simulink model "seti_ct_xaui"  (Simulink 6.2)
settings: Solver=ode45  StartTime=0.0  StopTime=10  RelTol=1e-3
undefined symbols (not defined in the file): bigColBits, bigRowBits, smallColBits, smallRowBits
libraries: xbsIndex_r3 x520, xps_library x31, casper_library x10, fft_library x1
(part 2 of 4)

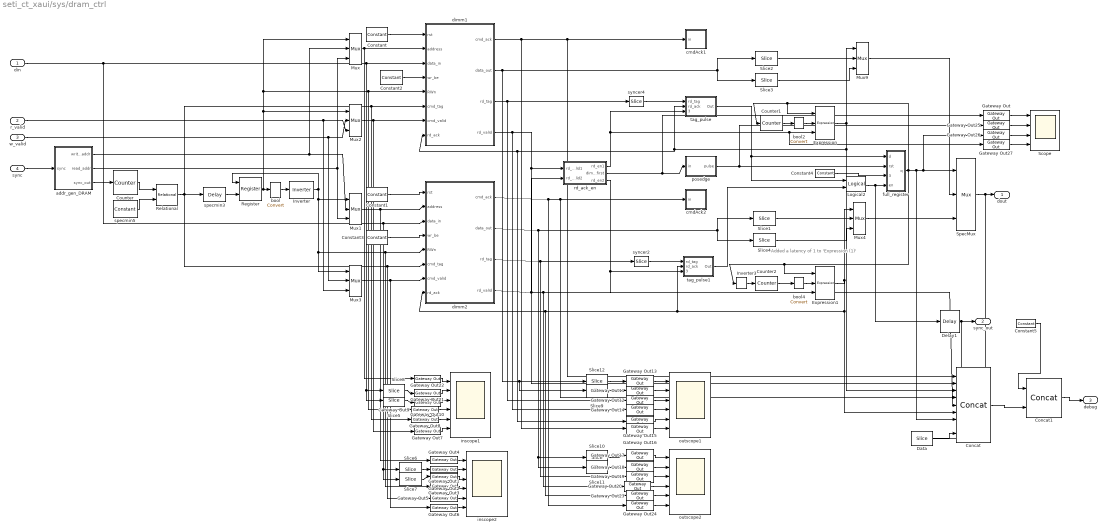
== system seti_ct_xaui/sys/dram_ctrl ==
  note: Added a latency
      | of 1 to 'Expression (1)'
  din : Inport  Port=1  LatchInput=off
  r_valid : Inport  Port=2  LatchInput=off
  w_valid : Inport  Port=3  LatchInput=off
  sync : Inport  Port=4  LatchInput=off
  Concat : xbsIndex_r3/Concat  num_inputs=9  explicit_period=off  period=1  dbl_ovrd=off
  Concat1 : xbsIndex_r3/Concat  num_inputs=2  explicit_period=off  period=1  dbl_ovrd=off
  Constant : xbsIndex_r3/Constant  const=0  equ=P=C  arith_type=Boolean  n_bits=1  bin_pt=0  opselect=C  inp2=PCIN>>17  opr=+  inp1=P  carry=CIN  iostate=0  explicit_period=on  period=1  dbl_ovrd=off
  Constant1 : xbsIndex_r3/Constant  const=0  equ=P=C  arith_type=Boolean  n_bits=1  bin_pt=0  opselect=C  inp2=PCIN>>17  opr=+  inp1=P  carry=CIN  iostate=0  explicit_period=on  period=1  dbl_ovrd=off
  Constant2 : xbsIndex_r3/Constant  const=2^18-1  equ=P=C  arith_type=Unsigned  n_bits=18  bin_pt=0  opselect=C  inp2=PCIN>>17  opr=+  inp1=P  carry=CIN  iostate=0  explicit_period=on  period=1  dbl_ovrd=off
  Constant3 : xbsIndex_r3/Constant  const=2^18-1  equ=P=C  arith_type=Unsigned  n_bits=18  bin_pt=0  opselect=C  inp2=PCIN>>17  opr=+  inp1=P  carry=CIN  iostate=0  explicit_period=on  period=1  dbl_ovrd=off
  Constant4 : xbsIndex_r3/Constant  const=0  equ=P=C  arith_type=Boolean  n_bits=1  bin_pt=0  opselect=C  inp2=PCIN>>17  opr=+  inp1=P  carry=CIN  iostate=0  explicit_period=off  period=1  dbl_ovrd=off
  Constant5 : xbsIndex_r3/Constant  const=0  equ=P=C  arith_type=Unsigned  n_bits=8  bin_pt=0  opselect=C  inp2=PCIN>>17  opr=+  inp1=P  carry=CIN  iostate=0  explicit_period=off  period=1  dbl_ovrd=off
  Counter : xbsIndex_r3/Counter  cnt_type=Free Running  n_bits=spec_len + num_spec  bin_pt=0  arith_type=Unsigned  start_count=0  cnt_to=Inf  cnt_by_val=1  operation=Up  explicit_period=off  period=1  load_pin=off  rst=on  en=off  dbl_ovrd=off  show_param=off  use_rpm=on  gen_core=off
      settings: xl_area=[0, 0, 0, 0, 0, 0, 0]
  Counter1 : xbsIndex_r3/Counter  cnt_type=Free Running  n_bits=1  bin_pt=0  arith_type=Unsigned  start_count=0  cnt_to=Inf  cnt_by_val=1  operation=Up  explicit_period=off  period=1  load_pin=off  rst=on  en=off  dbl_ovrd=off  show_param=off  use_rpm=on  gen_core=off
      settings: xl_area=[0, 0, 0, 0, 0, 0, 0]
  Counter2 : xbsIndex_r3/Counter  cnt_type=Free Running  n_bits=1  bin_pt=0  arith_type=Unsigned  start_count=0  cnt_to=Inf  cnt_by_val=1  operation=Up  explicit_period=off  period=1  load_pin=off  rst=on  en=off  dbl_ovrd=off  show_param=off  use_rpm=on  gen_core=off
      settings: xl_area=[0, 0, 0, 0, 0, 0, 0]
  Data : xbsIndex_r3/Slice  mode=Lower Bit Location + Width  nbits=16  bit1=0  base1=MSB of Input  bit0=0  base0=LSB of Input  boolean_output=off  explicit_period=off  period=1  dbl_ovrd=off
  Delay1 : xbsIndex_r3/Delay  latency=1  reg_retiming=off  explicit_period=off  period=1  en=off  accept_only_valid=off  init_zero=on  dbl_ovrd=off  show_param=off
      settings: xl_area=[0, 0, 0, 0, 0, 0, 0]
  Expression : xbsIndex_r3/Expression  expression=~a & b & c  precision=Full  arith_type=Unsigned  n_bits=8  bin_pt=2  align_bp=on  latency=1  explicit_period=off  period=1  en=off  dbl_ovrd=off  show_param=off
      settings: xl_area=[0, 0, 0, 0, 0, 0, 0]
  Expression1 : xbsIndex_r3/Expression  expression=a & b & c  precision=Full  arith_type=Unsigned  n_bits=8  bin_pt=2  align_bp=on  latency=1  explicit_period=off  period=1  en=off  dbl_ovrd=off  show_param=off
      settings: xl_area=[0, 0, 0, 0, 0, 0, 0]
  Gateway Out{,25..27} (4 alike) : xbsIndex_r3/Gateway Out  output_type=Double  nbits=8  bin_pt=6  arith_type=Boolean  quantization=Truncate  overflow=Wrap  hdl_port=on  timing_constraint=None  locs_specified=off  LOCs={}  needs_fixed_name=off  show_param=off
      settings: xl_area=[0, 0, 0, 0, 0, 0, 0]
  Gateway Out{1..24} (24 alike) : xbsIndex_r3/Gateway Out  output_type=Double  nbits=8  bin_pt=6  arith_type=Boolean  quantization=Truncate  overflow=Wrap  hdl_port=off  timing_constraint=None  locs_specified=off  LOCs={}  needs_fixed_name=off  show_param=off
      settings: xl_area=[0, 0, 0, 0, 0, 0, 0]
  Inverter : xbsIndex_r3/Inverter  latency=0  explicit_period=off  period=1  en=off  dbl_ovrd=off  show_param=off
      settings: xl_area=[0, 0, 0, 0, 0, 0, 0]
  Inverter3 : xbsIndex_r3/Inverter  latency=0  explicit_period=off  period=1  en=off  dbl_ovrd=off  show_param=off
      settings: xl_area=[0, 0, 0, 0, 0, 0, 0]
  Logical2 : xbsIndex_r3/Logical  logical_function=OR  inputs=2  precision=Full  arith_type=Unsigned  n_bits=8  bin_pt=2  align_bp=on  latency=0  explicit_period=off  period=1  en=off  dbl_ovrd=off  show_param=off
      settings: xl_area=[0, 0, 0, 0, 0, 0, 0]
  Mux{,1..4,9} (6 alike) : xbsIndex_r3/Mux  inputs=2  precision=Full  arith_type="Signed  (2's comp)"  n_bits=8  bin_pt=2  quantization=Truncate  overflow=Wrap  latency=0  explicit_period=off  period=1  en=off  dbl_ovrd=off  show_param=off  mux_type=off  use_rpm=off  gen_core=off
      settings: xl_area=[0, 0, 0, 0, 0, 0, 0]
  Register : xbsIndex_r3/Register  init=0  reg_only_valid=off  explicit_period=off  period=1  rst=off  en=on  out_en=off  dbl_ovrd=off  show_param=off
      settings: xl_area=[0, 0, 0, 0, 0, 0, 0]
  Relational : xbsIndex_r3/Relational  mode=a=b  latency=1  explicit_period=off  period=1  en=off  dbl_ovrd=off  show_param=off
      settings: xl_area=[0, 0, 0, 0, 0, 0, 0]
  Scope : Scope  NumInputPorts=4
      settings: YMin=-5~-5~-5~-5  YMax=5~5~5~5  SaveName=ScopeData11
  Slice{1..2,5,7,9,11} (6 alike) : xbsIndex_r3/Slice  mode=Lower Bit Location + Width  nbits=72  bit1=0  base1=MSB of Input  bit0=0  base0=LSB of Input  boolean_output=off  explicit_period=off  period=1  dbl_ovrd=off
  Slice{3..4,6,8,10,12} (6 alike) : xbsIndex_r3/Slice  mode=Upper Bit Location + Width  nbits=72  bit1=0  base1=MSB of Input  bit0=0  base0=LSB of Input  boolean_output=off  explicit_period=off  period=1  dbl_ovrd=off
  SpecMux : xbsIndex_r3/Mux  inputs=2  precision=Full  arith_type="Signed  (2's comp)"  n_bits=8  bin_pt=2  quantization=Truncate  overflow=Wrap  latency=1  explicit_period=off  period=1  en=off  dbl_ovrd=off  show_param=off  mux_type=off  use_rpm=off  gen_core=off
      settings: xl_area=[0, 0, 0, 0, 0, 0, 0]
  addr_gen_DRAM : Subsystem  mask{numSpecs=2^num_spec, length=2^spec_len}
      mask prompts: numSpecs "Number of Spectrums?"; length "Length of Spectrum?"
      mask init:
      | address_gen_dram_mask;
  bool : xbsIndex_r3/Convert  arith_type=Boolean  n_bits=8  bin_pt=6  quantization=Truncate  overflow=Wrap  latency=0  explicit_period=on  period=1  dbl_ovrd=off  show_param=off  inserted_by_tool=off  pipeline=off
      settings: xl_area=[0, 0, 0, 0, 0, 0, 0]
  bool2 : xbsIndex_r3/Convert  arith_type=Boolean  n_bits=8  bin_pt=6  quantization=Truncate  overflow=Wrap  latency=0  explicit_period=on  period=1  dbl_ovrd=off  show_param=off  inserted_by_tool=off  pipeline=off
      settings: xl_area=[0, 0, 0, 0, 0, 0, 0]
  bool4 : xbsIndex_r3/Convert  arith_type=Boolean  n_bits=8  bin_pt=6  quantization=Truncate  overflow=Wrap  latency=0  explicit_period=on  period=1  dbl_ovrd=off  show_param=off  inserted_by_tool=off  pipeline=off
      settings: xl_area=[0, 0, 0, 0, 0, 0, 0]
  cmdAck1 : Subsystem
  cmdAck2 : Subsystem
  dimm1 : Subsystem  Tag=xps:dram  AncestorBlock=xps_library/dram  mask(dram){dimm=1, arith_type=Unsigned, bin_pt=0, ip_clock=200, sample_period=1, use_sim=on, bank_mgt=off, wide_data=off, half_burst=off}
      mask prompts: arith_type "Data Type"; bin_pt "Data binary point"; ip_clock "Datapath clock rate (MHz)"; sample_period "Sample period"; use_sim "Simulate DRAM using ModelSim"; bank_mgt "Enable bank management"; wide_data "Use wide data bus (288 bits)"; half_burst "Use half-burst"
      mask help:
      | Interface to 1GB DDR2 DIMMs on BEE2.
      |
      | To simulate using ModelSim, place a ModelSim block named 'ModelSim' (case-sensitive) in the top level of the design.
      mask init:
      | dram_mask;
      mask StyleString: popup(1|2|3|4),popup(Boolean|Unsigned|Signed  (2's comp)),edit,edit,edit,checkbox,checkbox,checkbox,checkbox
      mask CallbackString:
      | |||||||myname=gcb;
      | if strcmp(get_param(myname, 'wide_data'), 'off')
      |     set_param(myname, 'MaskEnables', {'on','on','on','on','on','on','on','on','on'});
      | else
      |     set_param(myname, 'half_burst', 'off');
      |     set_param(myname, 'MaskEnables', {'on','on','on','on','on','on','on','on','off'});
      | end|
  dimm2 : Subsystem  Tag=xps:dram  AncestorBlock=xps_library/dram  mask(dram){dimm=2, arith_type=Unsigned, bin_pt=0, ip_clock=200, sample_period=1, use_sim=on, bank_mgt=off, wide_data=off, half_burst=off}
      mask prompts: arith_type "Data Type"; bin_pt "Data binary point"; ip_clock "Datapath clock rate (MHz)"; sample_period "Sample period"; use_sim "Simulate DRAM using ModelSim"; bank_mgt "Enable bank management"; wide_data "Use wide data bus (288 bits)"; half_burst "Use half-burst"
      mask help:
      | Interface to 1GB DDR2 DIMMs on BEE2.
      |
      | To simulate using ModelSim, place a ModelSim block named 'ModelSim' (case-sensitive) in the top level of the design.
      mask init:
      | dram_mask;
      mask StyleString: popup(1|2|3|4),popup(Boolean|Unsigned|Signed  (2's comp)),edit,edit,edit,checkbox,checkbox,checkbox,checkbox
      mask CallbackString:
      | |||||||myname=gcb;
      | if strcmp(get_param(myname, 'wide_data'), 'off')
      |     set_param(myname, 'MaskEnables', {'on','on','on','on','on','on','on','on','on'});
      | else
      |     set_param(myname, 'half_burst', 'off');
      |     set_param(myname, 'MaskEnables', {'on','on','on','on','on','on','on','on','off'});
      | end|
  full_register : Subsystem  mask{num_bits=1, init_val=1}
      mask prompts: num_bits "Number of Bits"; init_val "Initial Value"
  inscope1 : Scope  NumInputPorts=6
      settings: TimeRange=45.11589403973511  YMin=0~0~0~0~0~-5  YMax=157.8428582181891~4.1454e+022~1~1~1~5  SaveName=ScopeData4
  inscope2 : Scope  NumInputPorts=6
      settings: TimeRange=45.11589403973511  YMin=0~0~0~0~0~-5  YMax=157.8428582181891~4.1454e+022~1~1~1~5  SaveName=ScopeData5
  outscope1 : Scope  NumInputPorts=6
      settings: TimeRange=45.11589403973511  YMin=1295~1295~-1~0.95~0~0  YMax=1335~1335~1~1.05~1~1  SaveName=ScopeData6
  outscope2 : Scope  NumInputPorts=6
      settings: TimeRange=45.11589403973511  YMin=-1~-1~-1~0~0~0  YMax=1~1~1~1~1~1  SaveName=ScopeData3
  posedge : Subsystem
  rd_ack_en : Subsystem  mask{ct_delay=ct_delay}
      mask prompts: ct_delay "Corner Turn Delay"
  specmin3 : xbsIndex_r3/Delay  latency=2  reg_retiming=off  explicit_period=off  period=1  en=off  accept_only_valid=off  init_zero=on  dbl_ovrd=off  show_param=off
      settings: xl_area=[0, 0, 0, 0, 0, 0, 0]
  specmin5 : xbsIndex_r3/Constant  const=2^(spec_len+num_spec) -5  equ=P=C  arith_type=Unsigned  n_bits=(spec_len+num_spec)  bin_pt=0  opselect=C  inp2=PCIN>>17  opr=+  inp1=P  carry=CIN  iostate=0  explicit_period=off  period=1  dbl_ovrd=off
  syncer2 : xbsIndex_r3/Slice  mode=Lower Bit Location + Width  nbits=1  bit1=0  base1=MSB of Input  bit0=0  base0=LSB of Input  boolean_output=on  explicit_period=on  period=1  dbl_ovrd=off
  syncer4 : xbsIndex_r3/Slice  mode=Lower Bit Location + Width  nbits=1  bit1=0  base1=MSB of Input  bit0=0  base0=LSB of Input  boolean_output=on  explicit_period=on  period=1  dbl_ovrd=off
  tag_pulse : Subsystem
  tag_pulse1 : Subsystem
  dout : Outport
  sync_out : Outport  Port=2
  debug : Outport  Port=3
  wires:
  Constant/1 -> dimm1/1(rst)
  Constant1/1 -> dimm2/1(rst)
  addr_gen_DRAM/2(read_addr) -> Mux/3, Mux1/3
  Mux/1 -> dimm1/2(address), Gateway Out22/1
  Mux1/1 -> dimm2/2(address), Gateway Out4/1
  Constant2/1 -> dimm1/4(wr_be)
  Constant3/1 -> dimm2/4(wr_be)
  addr_gen_DRAM/3(sync_out) -> Counter/1
  Register/1 -> Mux/1, dimm1/5(RWn), Gateway Out9/1, Mux2/1, bool/1
  Inverter/1 -> Mux1/1, Mux3/1, dimm2/5(RWn), Gateway Out3/1, Register/1
  Counter/1 -> Relational/1
  specmin5/1 -> Relational/2
  Relational/1 -> dimm1/6(cmd_tag), Gateway Out8/1, dimm2/6(cmd_tag), Gateway Out5/1, specmin3/1
  din/1 -> dimm1/3(data_in), Slice8/1, Slice5/1, dimm2/3(data_in), Slice6/1, Slice7/1
  sync/1 -> addr_gen_DRAM/1(sync)
  r_valid/1 -> Mux3/3, Mux2/3
  Mux2/1 -> dimm1/7(cmd_valid), Gateway Out7/1
  Mux3/1 -> dimm2/7(cmd_valid), Gateway Out6/1
  w_valid/1 -> Mux2/2, Mux3/2
  dimm1/3(rd_tag) -> syncer4/1, Gateway Out12/1
  dimm2/3(rd_tag) -> syncer2/1, Gateway Out19/1
  bool/1 -> Inverter/1
  Gateway Out22/1 -> inscope1/1
  Gateway Out21/1 -> inscope1/2
  Gateway Out10/1 -> inscope1/3
  Gateway Out9/1 -> inscope1/4
  Gateway Out8/1 -> inscope1/5
  Gateway Out4/1 -> inscope2/1
  Gateway Out1/1 -> inscope2/2
  Gateway Out2/1 -> inscope2/3
  Gateway Out3/1 -> inscope2/4
  Gateway Out5/1 -> inscope2/5
  Slice5/1 -> Gateway Out10/1
  Slice6/1 -> Gateway Out1/1
  Slice7/1 -> Gateway Out2/1
  Slice9/1 -> Gateway Out11/1
  Gateway Out12/1 -> outscope1/3
  Gateway Out14/1 -> outscope1/4
  Gateway Out15/1 -> outscope1/5
  Slice10/1 -> Gateway Out17/1
  Slice11/1 -> Gateway Out18/1
  Gateway Out13/1 -> outscope1/1
  Gateway Out11/1 -> outscope1/2
  dimm1/1(cmd_ack) -> Gateway Out16/1, cmdAck1/1(in), Concat/1
  dimm2/1(cmd_ack) -> Gateway Out24/1, cmdAck2/1(in), Concat/4
  dimm2/4(rd_valid) -> rd_ack_en/2(rd_valid2), Gateway Out20/1, Concat/5
  dimm1/4(rd_valid) -> Gateway Out14/1, rd_ack_en/1(rd_valid1), Concat/2
  dimm1/2(data_out) -> Slice12/1, Slice9/1, Slice2/1, Slice3/1
  dimm2/2(data_out) -> Slice10/1, Slice11/1, Slice4/1, Slice1/1
  Slice8/1 -> Gateway Out21/1
  Slice12/1 -> Gateway Out13/1
  Gateway Out7/1 -> inscope1/6
  Gateway Out16/1 -> outscope1/6
  Gateway Out19/1 -> outscope2/3
  Gateway Out20/1 -> outscope2/4
  Gateway Out23/1 -> outscope2/5
  Gateway Out17/1 -> outscope2/1
  Gateway Out18/1 -> outscope2/2
  Slice2/1 -> Mux9/2
  Slice3/1 -> Mux9/3
  Slice1/1 -> Mux4/2
  Slice4/1 -> Mux4/3
  Gateway Out6/1 -> inscope2/6
  Gateway Out24/1 -> outscope2/6
  Logical2/1 -> Delay1/1, full_register/4(en)
  tag_pulse1/1(Out) -> Logical2/2
  full_register/1(q) -> Inverter3/1, Expression1/1, Counter1/1, Expression/1, SpecMux/1, Gateway Out26/1, Concat/7
  Mux9/1 -> SpecMux/2
  Mux4/1 -> SpecMux/3
  SpecMux/1 -> dout/1, Data/1
  Inverter3/1 -> Counter2/1
  Expression/1 -> Mux9/1, dimm1/8(rd_ack), Gateway Out15/1, tag_pulse/2(rd_ack), Concat/3
  Expression1/1 -> Mux4/1, dimm2/8(rd_ack), Gateway Out23/1, tag_pulse1/2(rd_ack), Concat/6
  Counter1/1 -> bool2/1
  Counter2/1 -> bool4/1
  bool2/1 -> Expression/2
  bool4/1 -> Expression1/2
  addr_gen_DRAM/1(write_addr) -> Mux1/2, Mux/2
  syncer4/1 -> tag_pulse/1(rd_tag)
  syncer2/1 -> tag_pulse1/1(rd_tag)
  Delay1/1 -> sync_out/1, Concat/8
  rd_ack_en/1(rd_en1) -> tag_pulse/3(rd_valid), Expression/3, Gateway Out27/1
  rd_ack_en/3(rd_en2) -> tag_pulse1/3(rd_valid), Expression1/3
  rd_ack_en/2(dimm1_first) -> posedge/1(in), Gateway Out/1
  tag_pulse/1(Out) -> Logical2/1, full_register/1(d)
  posedge/1(pulse) -> Gateway Out25/1, full_register/2(rst)
  Gateway Out/1 -> Scope/1
  Gateway Out25/1 -> Scope/2
  Gateway Out26/1 -> Scope/3
  Gateway Out27/1 -> Scope/4
  Constant4/1 -> full_register/3(set)
  specmin3/1 -> Register/2
  Data/1 -> Concat/9
  Concat/1 -> Concat1/2
  Concat1/1 -> debug/1
  Constant5/1 -> Concat1/1

== system seti_ct_xaui/sys/dram_in ==
  din : Inport  Port=1  LatchInput=off
  sync : Inport  Port=2  LatchInput=off
  Concat : xbsIndex_r3/Concat  num_inputs=2  explicit_period=off  period=1  dbl_ovrd=off
  Counter : xbsIndex_r3/Counter  cnt_type=Free Running  n_bits=2  bin_pt=0  arith_type=Unsigned  start_count=0  cnt_to=Inf  cnt_by_val=1  operation=Up  explicit_period=off  period=1  load_pin=off  rst=on  en=on  dbl_ovrd=off  show_param=off  use_rpm=on  gen_core=off
      settings: xl_area=[0, 0, 0, 0, 0, 0, 0]
  Delay1 : xbsIndex_r3/Delay  latency=1  reg_retiming=off  explicit_period=off  period=1  en=off  accept_only_valid=off  init_zero=on  dbl_ovrd=off  show_param=off
      settings: xl_area=[0, 0, 0, 0, 0, 0, 0]
  Delay2 : xbsIndex_r3/Delay  latency=1  reg_retiming=off  explicit_period=off  period=1  en=off  accept_only_valid=off  init_zero=on  dbl_ovrd=off  show_param=off
      settings: xl_area=[0, 0, 0, 0, 0, 0, 0]
  Delay3 : xbsIndex_r3/Delay  latency=2  reg_retiming=off  explicit_period=off  period=1  en=off  accept_only_valid=off  init_zero=on  dbl_ovrd=off  show_param=off
      settings: xl_area=[0, 0, 0, 0, 0, 0, 0]
  Gateway Out1 : xbsIndex_r3/Gateway Out  output_type=Double  nbits=8  bin_pt=6  arith_type=Boolean  quantization=Truncate  overflow=Wrap  hdl_port=off  timing_constraint=None  locs_specified=off  LOCs={}  needs_fixed_name=off  show_param=off
      settings: xl_area=[0, 0, 0, 0, 0, 0, 0]
  Gateway Out5 : xbsIndex_r3/Gateway Out  output_type=Double  nbits=8  bin_pt=6  arith_type=Boolean  quantization=Truncate  overflow=Wrap  hdl_port=off  timing_constraint=None  locs_specified=off  LOCs={}  needs_fixed_name=off  show_param=off
      settings: xl_area=[0, 0, 0, 0, 0, 0, 0]
  HighBit : xbsIndex_r3/Slice  mode=Upper Bit Location + Width  nbits=1  bit1=0  base1=MSB of Input  bit0=0  base0=LSB of Input  boolean_output=on  explicit_period=off  period=1  dbl_ovrd=off
  LowBit : xbsIndex_r3/Slice  mode=Lower Bit Location + Width  nbits=1  bit1=0  base1=MSB of Input  bit0=0  base0=LSB of Input  boolean_output=on  explicit_period=off  period=1  dbl_ovrd=off
  Mux : xbsIndex_r3/Mux  inputs=2  precision=Full  arith_type="Signed  (2's comp)"  n_bits=8  bin_pt=2  quantization=Truncate  overflow=Wrap  latency=0  explicit_period=off  period=1  en=off  dbl_ovrd=off  show_param=off  mux_type=off  use_rpm=off  gen_core=off
      settings: xl_area=[0, 0, 0, 0, 0, 0, 0]
  Register : xbsIndex_r3/Register  init=0  reg_only_valid=off  explicit_period=off  period=1  rst=off  en=on  out_en=off  dbl_ovrd=off  show_param=off
      settings: xl_area=[0, 0, 0, 0, 0, 0, 0]
  Scope : Scope  NumInputPorts=2
      settings: YMin=-5~-5  YMax=5~5  SaveName=ScopeData8
  dbuf_transpose : Subsystem  AncestorBlock=reorder_library/dbuf_transpose  mask{Rows=spec_len, Cols=2, bram_latency=2}
      mask prompts: Rows "Rows of Matrix (data written in): (2^?)"; Cols "Cols of Matrix (data read out): (2^?)"; bram_latency "BRAM Latency"
  is2 : xbsIndex_r3/Expression  expression=~a & b  precision=Full  arith_type=Unsigned  n_bits=8  bin_pt=2  align_bp=on  latency=0  explicit_period=off  period=1  en=off  dbl_ovrd=off  show_param=off
      settings: xl_area=[0, 0, 0, 0, 0, 0, 0]
  dout : Outport
  r_valid : Outport  Port=2
  w_valid : Outport  Port=3
  sync_out : Outport  Port=4
  wires:
  dbuf_transpose/2(sync_out) -> Counter/1, Register/1, Delay3/1, Register/2, Gateway Out1/1
  Delay1/1 -> Concat/2
  dbuf_transpose/1(dout) -> Delay1/1, Concat/1, Gateway Out5/1
  sync/1 -> dbuf_transpose/2(sync)
  din/1 -> dbuf_transpose/1(din)
  Counter/1 -> HighBit/1, LowBit/1
  Mux/1 -> dout/1
  Concat/1 -> Mux/3, Delay2/1
  Delay2/1 -> Mux/2
  LowBit/1 -> Mux/1, is2/1
  Delay3/1 -> sync_out/1
  is2/1 -> r_valid/1
  HighBit/1 -> is2/2, w_valid/1
  Register/1 -> Counter/2
  Gateway Out5/1 -> Scope/1
  Gateway Out1/1 -> Scope/2

== system seti_ct_xaui/sys/pack ==
  sync : Inport  Port=1  LatchInput=off
  data : Inport  Port=2  LatchInput=off
  Concat : xbsIndex_r3/Concat  num_inputs=4  explicit_period=on  period=1  dbl_ovrd=off
  Constant10 : xbsIndex_r3/Constant  const=0  equ=P=C  arith_type=Unsigned  n_bits=1  bin_pt=0  opselect=C  inp2=PCIN>>17  opr=+  inp1=P  carry=CIN  iostate=0  explicit_period=on  period=1  dbl_ovrd=off
  Convert3 : xbsIndex_r3/Convert  arith_type=Unsigned  n_bits=1  bin_pt=0  quantization=Truncate  overflow=Wrap  latency=1  explicit_period=on  period=1  dbl_ovrd=off  show_param=off  inserted_by_tool=off  pipeline=off
      settings: xl_area=[0, 0, 0, 0, 0, 0, 0]
  Convert4 : xbsIndex_r3/Convert  arith_type="Signed  (2's comp)"  n_bits=15  bin_pt=14  quantization=Truncate  overflow=Wrap  latency=1  explicit_period=on  period=1  dbl_ovrd=off  show_param=off  inserted_by_tool=off  pipeline=off
      settings: xl_area=[0, 0, 0, 0, 0, 0, 0]
  Convert5 : xbsIndex_r3/Convert  arith_type="Signed  (2's comp)"  n_bits=15  bin_pt=14  quantization=Truncate  overflow=Wrap  latency=1  explicit_period=on  period=1  dbl_ovrd=off  show_param=off  inserted_by_tool=off  pipeline=off
      settings: xl_area=[0, 0, 0, 0, 0, 0, 0]
  Reinterpret : xbsIndex_r3/Reinterpret  force_arith_type=on  arith_type=Unsigned  force_bin_pt=on  bin_pt=0  force_valid=on
  Reinterpret1 : xbsIndex_r3/Reinterpret  force_arith_type=on  arith_type=Unsigned  force_bin_pt=on  bin_pt=0  force_valid=on
  c_to_ri : casper_library/Misc/c_to_ri  n_bits=18  bin_pt=17
      settings: AttributesFormatString=18_17 r/i
  out : Outport
  wires:
  Constant10/1 -> Concat/1
  c_to_ri/1 -> Convert4/1
  c_to_ri/2 -> Convert5/1
  Convert3/1 -> Concat/2
  Convert4/1 -> Reinterpret/1
  Reinterpret/1 -> Concat/3
  sync/1 -> Convert3/1
  Concat/1 -> out/1
  data/1 -> c_to_ri/1
  Convert5/1 -> Reinterpret1/1
  Reinterpret1/1 -> Concat/4

== system seti_ct_xaui/sys/pack1 ==
  sync : Inport  Port=1  LatchInput=off
  data : Inport  Port=2  LatchInput=off
  Concat : xbsIndex_r3/Concat  num_inputs=4  explicit_period=on  period=1  dbl_ovrd=off
  Constant10 : xbsIndex_r3/Constant  const=0  equ=P=C  arith_type=Unsigned  n_bits=1  bin_pt=0  opselect=C  inp2=PCIN>>17  opr=+  inp1=P  carry=CIN  iostate=0  explicit_period=on  period=1  dbl_ovrd=off
  Convert3 : xbsIndex_r3/Convert  arith_type=Unsigned  n_bits=1  bin_pt=0  quantization=Truncate  overflow=Wrap  latency=1  explicit_period=on  period=1  dbl_ovrd=off  show_param=off  inserted_by_tool=off  pipeline=off
      settings: xl_area=[0, 0, 0, 0, 0, 0, 0]
  Convert4 : xbsIndex_r3/Convert  arith_type="Signed  (2's comp)"  n_bits=15  bin_pt=14  quantization=Truncate  overflow=Wrap  latency=1  explicit_period=on  period=1  dbl_ovrd=off  show_param=off  inserted_by_tool=off  pipeline=off
      settings: xl_area=[0, 0, 0, 0, 0, 0, 0]
  Convert5 : xbsIndex_r3/Convert  arith_type="Signed  (2's comp)"  n_bits=15  bin_pt=14  quantization=Truncate  overflow=Wrap  latency=1  explicit_period=on  period=1  dbl_ovrd=off  show_param=off  inserted_by_tool=off  pipeline=off
      settings: xl_area=[0, 0, 0, 0, 0, 0, 0]
  Reinterpret : xbsIndex_r3/Reinterpret  force_arith_type=on  arith_type=Unsigned  force_bin_pt=on  bin_pt=0  force_valid=on
  Reinterpret1 : xbsIndex_r3/Reinterpret  force_arith_type=on  arith_type=Unsigned  force_bin_pt=on  bin_pt=0  force_valid=on
  c_to_ri : casper_library/Misc/c_to_ri  n_bits=18  bin_pt=17
      settings: AttributesFormatString=18_17 r/i
  out : Outport
  wires:
  Reinterpret1/1 -> Concat/4
  Convert5/1 -> Reinterpret1/1
  data/1 -> c_to_ri/1
  Concat/1 -> out/1
  sync/1 -> Convert3/1
  Reinterpret/1 -> Concat/3
  Convert4/1 -> Reinterpret/1
  Convert3/1 -> Concat/2
  c_to_ri/2 -> Convert5/1
  c_to_ri/1 -> Convert4/1
  Constant10/1 -> Concat/1

== system seti_ct_xaui/sys/split ==
  In1 : Inport  Port=1  LatchInput=off
  Convert : xbsIndex_r3/Convert  arith_type="Signed  (2's comp)"  n_bits=18  bin_pt=17  quantization=Truncate  overflow=Wrap  latency=0  explicit_period=on  period=1  dbl_ovrd=off  show_param=off  inserted_by_tool=off  pipeline=off
      settings: xl_area=[0, 0, 0, 0, 0, 0, 0]
  Convert1 : xbsIndex_r3/Convert  arith_type="Signed  (2's comp)"  n_bits=18  bin_pt=17  quantization=Truncate  overflow=Wrap  latency=0  explicit_period=on  period=1  dbl_ovrd=off  show_param=off  inserted_by_tool=off  pipeline=off
      settings: xl_area=[0, 0, 0, 0, 0, 0, 0]
  Slice5 : xbsIndex_r3/Slice  mode=Lower Bit Location + Width  nbits=15  bit1=0  base1=MSB of Input  bit0=0  base0=LSB of Input  boolean_output=off  explicit_period=on  period=1  dbl_ovrd=off
  Slice6 : xbsIndex_r3/Slice  mode=Lower Bit Location + Width  nbits=15  bit1=0  base1=MSB of Input  bit0=15  base0=LSB of Input  boolean_output=off  explicit_period=on  period=1  dbl_ovrd=off
  Slice9 : xbsIndex_r3/Slice  mode=Lower Bit Location + Width  nbits=1  bit1=0  base1=MSB of Input  bit0=30  base0=LSB of Input  boolean_output=on  explicit_period=on  period=1  dbl_ovrd=off
  ri_to_c : casper_library/Misc/ri_to_c
  sync : Outport
  data : Outport  Port=2
  wires:
  In1/1 -> Slice5/1, Slice6/1, Slice9/1
  Slice6/1 -> Convert/1
  Slice5/1 -> Convert1/1
  Convert/1 -> ri_to_c/1
  Convert1/1 -> ri_to_c/2
  Slice9/1 -> sync/1
  ri_to_c/1 -> data/1

== system seti_ct_xaui/sys/trig_delay ==
  data_in : Inport  Port=1  LatchInput=off
  trig_in : Inport  Port=2  LatchInput=off
  delay : Inport  Port=3  LatchInput=off
  Constant : xbsIndex_r3/Constant  const=1  equ=P=C  arith_type=Boolean  n_bits=32  bin_pt=0  opselect=C  inp2=PCIN>>17  opr=+  inp1=P  carry=CIN  iostate=0  explicit_period=on  period=1  dbl_ovrd=off
  Counter : xbsIndex_r3/Counter  cnt_type=Free Running  n_bits=32  bin_pt=0  arith_type=Unsigned  start_count=0  cnt_to=Inf  cnt_by_val=1  operation=Up  explicit_period=on  period=1  load_pin=off  rst=on  en=on  dbl_ovrd=off  show_param=off  use_rpm=on  gen_core=off
      settings: xl_area=[0, 0, 0, 0, 0, 0, 0]
  Delay : xbsIndex_r3/Delay  latency=2  reg_retiming=off  explicit_period=on  period=1  en=off  accept_only_valid=off  init_zero=on  dbl_ovrd=off  show_param=off
      settings: xl_area=[0, 0, 0, 0, 0, 0, 0]
  Gateway Out : xbsIndex_r3/Gateway Out  output_type=Double  nbits=8  bin_pt=6  arith_type=Boolean  quantization=Truncate  overflow=Wrap  hdl_port=on  timing_constraint=None  locs_specified=off  LOCs={}  needs_fixed_name=off  show_param=off
      settings: xl_area=[0, 0, 0, 0, 0, 0, 0]
  Gateway Out1 : xbsIndex_r3/Gateway Out  output_type=Double  nbits=8  bin_pt=6  arith_type=Boolean  quantization=Truncate  overflow=Wrap  hdl_port=on  timing_constraint=None  locs_specified=off  LOCs={}  needs_fixed_name=off  show_param=off
      settings: xl_area=[0, 0, 0, 0, 0, 0, 0]
  Register : xbsIndex_r3/Register  init=0  reg_only_valid=off  explicit_period=on  period=1  rst=on  en=on  out_en=off  dbl_ovrd=off  show_param=off
      settings: xl_area=[0, 0, 0, 0, 0, 0, 0]
  Relational : xbsIndex_r3/Relational  mode=a=b  latency=1  explicit_period=on  period=1  en=on  dbl_ovrd=off  show_param=off
      settings: xl_area=[0, 0, 0, 0, 0, 0, 0]
  Scope : Scope  NumInputPorts=2
      settings: YMin=-5~-5  YMax=5~5
  posedge : casper_library/Misc/posedge  Tag=Rising Edge Detector
  data_out : Outport
  trig_out : Outport  Port=2
  wires:
  delay/1 -> Relational/1
  trig_in/1 -> Register/3, Gateway Out1/1
  Constant/1 -> Register/1
  Relational/1 -> Register/2, Counter/1, Gateway Out/1, posedge/1
  Register/1 -> Counter/2, Relational/3
  Counter/1 -> Relational/2
  Gateway Out/1 -> Scope/1
  Gateway Out1/1 -> Scope/2
  data_in/1 -> Delay/1
  Delay/1 -> data_out/1
  posedge/1 -> trig_out/1

== system seti_ct_xaui/sys/trig_delay1 ==
  data_in : Inport  Port=1  LatchInput=off
  trig_in : Inport  Port=2  LatchInput=off
  delay : Inport  Port=3  LatchInput=off
  Constant : xbsIndex_r3/Constant  const=1  equ=P=C  arith_type=Boolean  n_bits=32  bin_pt=0  opselect=C  inp2=PCIN>>17  opr=+  inp1=P  carry=CIN  iostate=0  explicit_period=on  period=1  dbl_ovrd=off
  Counter : xbsIndex_r3/Counter  cnt_type=Free Running  n_bits=32  bin_pt=0  arith_type=Unsigned  start_count=0  cnt_to=Inf  cnt_by_val=1  operation=Up  explicit_period=on  period=1  load_pin=off  rst=on  en=on  dbl_ovrd=off  show_param=off  use_rpm=on  gen_core=off
      settings: xl_area=[0, 0, 0, 0, 0, 0, 0]
  Delay : xbsIndex_r3/Delay  latency=2  reg_retiming=off  explicit_period=on  period=1  en=off  accept_only_valid=off  init_zero=on  dbl_ovrd=off  show_param=off
      settings: xl_area=[0, 0, 0, 0, 0, 0, 0]
  Gateway Out : xbsIndex_r3/Gateway Out  output_type=Double  nbits=8  bin_pt=6  arith_type=Boolean  quantization=Truncate  overflow=Wrap  hdl_port=on  timing_constraint=None  locs_specified=off  LOCs={}  needs_fixed_name=off  show_param=off
      settings: xl_area=[0, 0, 0, 0, 0, 0, 0]
  Gateway Out1 : xbsIndex_r3/Gateway Out  output_type=Double  nbits=8  bin_pt=6  arith_type=Boolean  quantization=Truncate  overflow=Wrap  hdl_port=on  timing_constraint=None  locs_specified=off  LOCs={}  needs_fixed_name=off  show_param=off
      settings: xl_area=[0, 0, 0, 0, 0, 0, 0]
  Register : xbsIndex_r3/Register  init=0  reg_only_valid=off  explicit_period=on  period=1  rst=on  en=on  out_en=off  dbl_ovrd=off  show_param=off
      settings: xl_area=[0, 0, 0, 0, 0, 0, 0]
  Relational : xbsIndex_r3/Relational  mode=a=b  latency=1  explicit_period=on  period=1  en=on  dbl_ovrd=off  show_param=off
      settings: xl_area=[0, 0, 0, 0, 0, 0, 0]
  Scope : Scope  NumInputPorts=2
      settings: YMin=-5~-5  YMax=5~5
  posedge : casper_library/Misc/posedge  Tag=Rising Edge Detector
  data_out : Outport
  trig_out : Outport  Port=2
  wires:
  delay/1 -> Relational/1
  trig_in/1 -> Register/3, Gateway Out1/1
  Constant/1 -> Register/1
  Relational/1 -> Register/2, Counter/1, Gateway Out/1, posedge/1
  Register/1 -> Counter/2, Relational/3
  Counter/1 -> Relational/2
  Gateway Out/1 -> Scope/1
  Gateway Out1/1 -> Scope/2
  data_in/1 -> Delay/1
  Delay/1 -> data_out/1
  posedge/1 -> trig_out/1

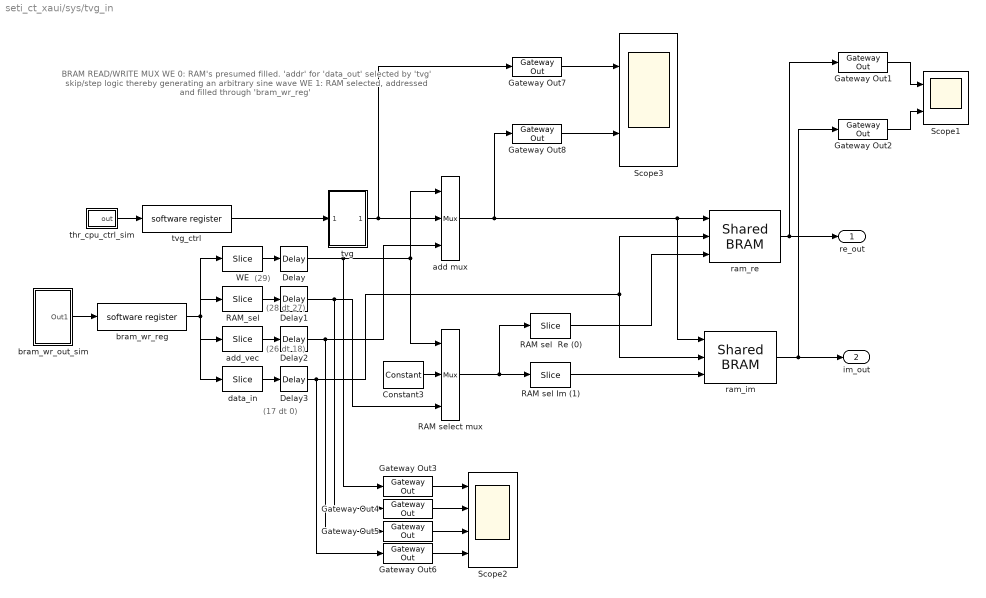
== system seti_ct_xaui/sys/tvg_in ==
  note: BRAM READ/WRITE MUX
      | WE 0: RAM's presumed filled.
      | 'addr' for 'data_out' selected
      | by 'tvg' skip/step logic thereby
      | generating an arbitrary sine wave
      | WE 1: RAM selected, addressed
      | and filled through
      | 'bram_wr_reg'
  note: (29)
  note: (28 dt 27)
  note: (17 dt 0)
  note: (26 dt 18)
  Constant3 : xbsIndex_r3/Constant  const=0  equ=P=C  arith_type=Unsigned  n_bits=4  bin_pt=0  opselect=C  inp2=PCIN>>17  opr=+  inp1=P  carry=CIN  iostate=0  explicit_period=on  period=1  dbl_ovrd=off
  Delay{,1..3} (4 alike) : xbsIndex_r3/Delay  latency=1  reg_retiming=off  explicit_period=on  period=1  en=off  accept_only_valid=off  init_zero=on  dbl_ovrd=off  show_param=off
      settings: xl_area=[0, 0, 0, 0, 0, 0, 0]
  Gateway Out{1..8} (8 alike) : xbsIndex_r3/Gateway Out  output_type=Double  nbits=8  bin_pt=6  arith_type=Boolean  quantization=Truncate  overflow=Wrap  hdl_port=on  timing_constraint=None  locs_specified=off  LOCs={}  needs_fixed_name=off  show_param=off
      settings: xl_area=[0, 0, 0, 0, 0, 0, 0]
  RAM sel  Re (0) : xbsIndex_r3/Slice  mode=Lower Bit Location + Width  nbits=1  bit1=0  base1=MSB of Input  bit0=0  base0=LSB of Input  boolean_output=on  explicit_period=on  period=1  dbl_ovrd=off
  RAM sel Im (1) : xbsIndex_r3/Slice  mode=Lower Bit Location + Width  nbits=1  bit1=0  base1=MSB of Input  bit0=1  base0=LSB of Input  boolean_output=on  explicit_period=on  period=1  dbl_ovrd=off
  RAM select mux : xbsIndex_r3/Mux  inputs=2  precision=Full  arith_type="Signed  (2's comp)"  n_bits=8  bin_pt=2  quantization=Truncate  overflow=Wrap  latency=0  explicit_period=on  period=1  en=off  dbl_ovrd=off  show_param=off  mux_type=off  use_rpm=off  gen_core=off
      settings: xl_area=[0, 0, 0, 0, 0, 0, 0]
  RAM_sel : xbsIndex_r3/Slice  mode=Lower Bit Location + Width  nbits=2  bit1=10  base1=MSB of Input  bit0=27  base0=LSB of Input  boolean_output=off  explicit_period=on  period=1  dbl_ovrd=off
  Scope1 : Scope  NumInputPorts=2
      settings: YMin=-5~-5  YMax=5~5  SaveName=ScopeData2
  Scope2 : Scope  NumInputPorts=4
      settings: YMin=-5~-5~-5~-5  YMax=5~5~5~5
  Scope3 : Scope  NumInputPorts=2
      settings: YMin=-5~-5  YMax=5~5  SaveName=ScopeData3
  WE : xbsIndex_r3/Slice  mode=Lower Bit Location + Width  nbits=1  bit1=10  base1=MSB of Input  bit0=29  base0=LSB of Input  boolean_output=off  explicit_period=on  period=1  dbl_ovrd=off
  add mux : xbsIndex_r3/Mux  inputs=2  precision=Full  arith_type="Signed  (2's comp)"  n_bits=8  bin_pt=2  quantization=Truncate  overflow=Wrap  latency=0  explicit_period=on  period=1  en=off  dbl_ovrd=off  show_param=off  mux_type=off  use_rpm=off  gen_core=off
      settings: xl_area=[0, 0, 0, 0, 0, 0, 0]
  add_vec : xbsIndex_r3/Slice  mode=Lower Bit Location + Width  nbits=9  bit1=0  base1=MSB of Input  bit0=18  base0=LSB of Input  boolean_output=off  explicit_period=on  period=1  dbl_ovrd=off
  bram_wr_out_sim : Subsystem  mask{we_enable=0, ram_sel=3, add_vec=512, data_in=32}
      mask prompts: we_enable "Write enable"; ram_sel "RAM selector (1 = Re; 2 = Im; 3 = both)"; add_vec "RAM address"; data_in "Data in"
  bram_wr_reg : xps_library/software register  Tag=xps:sw_reg  io_dir=From Processor  arith_type=Unsigned  bitwidth=32  bin_pt=0  sample_period=1  gw_name=seti_ct_xaui_sys_tvg_in_bram_wr_reg_user_data_out
  data_in : xbsIndex_r3/Slice  mode=Lower Bit Location + Width  nbits=18  bit1=0  base1=MSB of Input  bit0=0  base0=LSB of Input  boolean_output=off  explicit_period=on  period=1  dbl_ovrd=off
  ram_im : xps_library/Shared BRAM  Tag=xps:bram  arith_type="Signed  (2's comp)"  addr_width=11  data_width=32  data_bin_pt=0  init_vals=[1:2^11]  sample_rate=1
  ram_re : xps_library/Shared BRAM  Tag=xps:bram  arith_type="Signed  (2's comp)"  addr_width=11  data_width=32  data_bin_pt=0  init_vals=[1:2^11]  sample_rate=1
  thr_cpu_ctrl_sim : Subsystem  mask{tvg_skip=1, tvg_stall=2, tvg_length=5}
      mask prompts: tvg_skip "Skip"; tvg_stall "Stall"; tvg_length "Length"
      mask help:
      | Mux Data for CT and FFT Syncs:
      |
      | 0 -> Interchip Connection
      | 1 -> User Generated External Sync
      | 2 -> Periodic Sync Generator
      | 3 -> Periodic Sync Generator (Same as 2)
      |
      | Mux Data for CT and FFT Inputs:
      |
      | 0 -> Interchip Connection
      | 1 -> Test Vector Generator (TVG)
      | 2 -> All Zeroes (0's)
      | 3 -> All Ones (1's)
  tvg : Subsystem  mask(Test Vector Generator(TVG)){tvg_skip=1, tvg_stall=1, tvg_length=512}
      mask prompts: tvg_skip "Skip"; tvg_stall "Stall"; tvg_length "Length"
  tvg_ctrl : xps_library/software register  Tag=xps:sw_reg  io_dir=From Processor  arith_type=Unsigned  bitwidth=32  bin_pt=0  sample_period=1  gw_name=seti_ct_xaui_sys_tvg_in_tvg_ctrl_user_data_out
  re_out : Outport
  im_out : Outport  Port=2
  wires:
  tvg_ctrl/1 -> tvg/1(In1)
  tvg/1(Out1) -> add mux/2, Gateway Out7/1
  Constant3/1 -> RAM select mux/2
  RAM select mux/1 -> RAM sel  Re (0)/1, RAM sel Im (1)/1
  RAM sel  Re (0)/1 -> ram_re/3
  WE/1 -> Delay/1
  Gateway Out1/1 -> Scope1/1
  Gateway Out2/1 -> Scope1/2
  thr_cpu_ctrl_sim/1(out) -> tvg_ctrl/1
  bram_wr_reg/1 -> data_in/1, add_vec/1, RAM_sel/1, WE/1
  add_vec/1 -> Delay2/1
  RAM_sel/1 -> Delay1/1
  add mux/1 -> ram_im/1, ram_re/1, Gateway Out8/1
  data_in/1 -> Delay3/1
  RAM sel Im (1)/1 -> ram_im/3
  ram_re/1 -> Gateway Out1/1, re_out/1
  ram_im/1 -> Gateway Out2/1, im_out/1
  bram_wr_out_sim/1(Out1) -> bram_wr_reg/1
  Gateway Out3/1 -> Scope2/1
  Gateway Out4/1 -> Scope2/2
  Gateway Out5/1 -> Scope2/3
  Gateway Out6/1 -> Scope2/4
  Delay/1 -> Gateway Out3/1, add mux/1, RAM select mux/1
  Delay1/1 -> Gateway Out4/1, RAM select mux/3
  Delay2/1 -> Gateway Out5/1, add mux/3
  Delay3/1 -> Gateway Out6/1, ram_re/2, ram_im/2
  Gateway Out7/1 -> Scope3/1
  Gateway Out8/1 -> Scope3/2

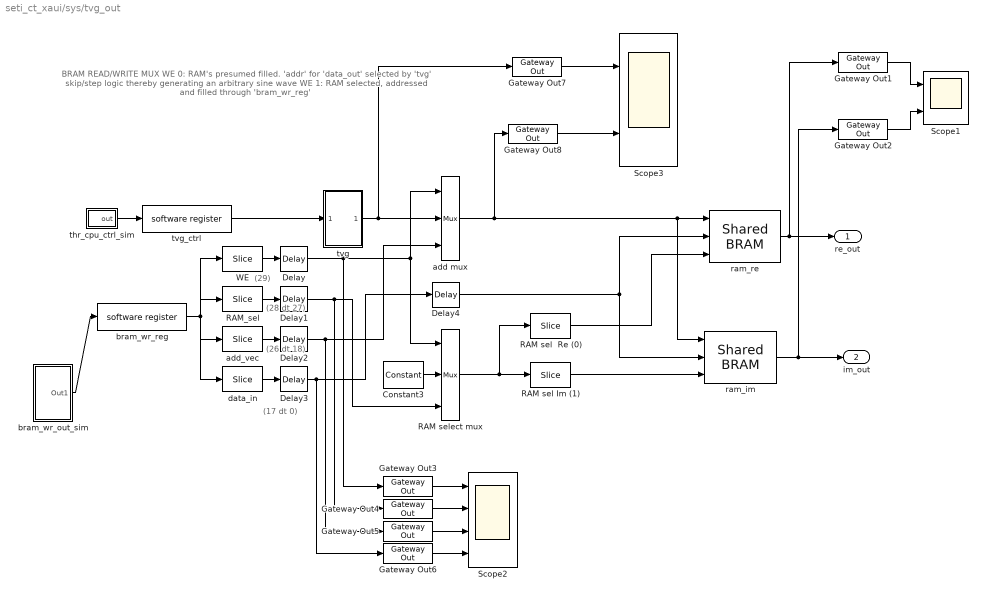
== system seti_ct_xaui/sys/tvg_out ==
  note: BRAM READ/WRITE MUX
      | WE 0: RAM's presumed filled.
      | 'addr' for 'data_out' selected
      | by 'tvg' skip/step logic thereby
      | generating an arbitrary sine wave
      | WE 1: RAM selected, addressed
      | and filled through
      | 'bram_wr_reg'
  note: (29)
  note: (28 dt 27)
  note: (17 dt 0)
  note: (26 dt 18)
  Constant3 : xbsIndex_r3/Constant  const=0  equ=P=C  arith_type=Unsigned  n_bits=4  bin_pt=0  opselect=C  inp2=PCIN>>17  opr=+  inp1=P  carry=CIN  iostate=0  explicit_period=on  period=1  dbl_ovrd=off
  Delay{,1..4} (5 alike) : xbsIndex_r3/Delay  latency=1  reg_retiming=off  explicit_period=on  period=1  en=off  accept_only_valid=off  init_zero=on  dbl_ovrd=off  show_param=off
      settings: xl_area=[0, 0, 0, 0, 0, 0, 0]
  Gateway Out{1..8} (8 alike) : xbsIndex_r3/Gateway Out  output_type=Double  nbits=8  bin_pt=6  arith_type=Boolean  quantization=Truncate  overflow=Wrap  hdl_port=on  timing_constraint=None  locs_specified=off  LOCs={}  needs_fixed_name=off  show_param=off
      settings: xl_area=[0, 0, 0, 0, 0, 0, 0]
  RAM sel  Re (0) : xbsIndex_r3/Slice  mode=Lower Bit Location + Width  nbits=1  bit1=0  base1=MSB of Input  bit0=0  base0=LSB of Input  boolean_output=on  explicit_period=on  period=1  dbl_ovrd=off
  RAM sel Im (1) : xbsIndex_r3/Slice  mode=Lower Bit Location + Width  nbits=1  bit1=0  base1=MSB of Input  bit0=1  base0=LSB of Input  boolean_output=on  explicit_period=on  period=1  dbl_ovrd=off
  RAM select mux : xbsIndex_r3/Mux  inputs=2  precision=Full  arith_type="Signed  (2's comp)"  n_bits=8  bin_pt=2  quantization=Truncate  overflow=Wrap  latency=1  explicit_period=on  period=1  en=off  dbl_ovrd=off  show_param=off  mux_type=off  use_rpm=off  gen_core=off
      settings: xl_area=[0, 0, 0, 0, 0, 0, 0]
  RAM_sel : xbsIndex_r3/Slice  mode=Lower Bit Location + Width  nbits=2  bit1=10  base1=MSB of Input  bit0=27  base0=LSB of Input  boolean_output=off  explicit_period=on  period=1  dbl_ovrd=off
  Scope1 : Scope  NumInputPorts=2
      settings: YMin=-5~-5  YMax=5~5  SaveName=ScopeData2
  Scope2 : Scope  NumInputPorts=4
      settings: YMin=-5~-5~-5~-5  YMax=5~5~5~5
  Scope3 : Scope  NumInputPorts=2
      settings: YMin=-5~-5  YMax=5~5  SaveName=ScopeData3
  WE : xbsIndex_r3/Slice  mode=Lower Bit Location + Width  nbits=1  bit1=10  base1=MSB of Input  bit0=29  base0=LSB of Input  boolean_output=off  explicit_period=on  period=1  dbl_ovrd=off
  add mux : xbsIndex_r3/Mux  inputs=2  precision=Full  arith_type="Signed  (2's comp)"  n_bits=8  bin_pt=2  quantization=Truncate  overflow=Wrap  latency=1  explicit_period=on  period=1  en=off  dbl_ovrd=off  show_param=off  mux_type=off  use_rpm=off  gen_core=off
      settings: xl_area=[0, 0, 0, 0, 0, 0, 0]
  add_vec : xbsIndex_r3/Slice  mode=Lower Bit Location + Width  nbits=9  bit1=0  base1=MSB of Input  bit0=18  base0=LSB of Input  boolean_output=off  explicit_period=on  period=1  dbl_ovrd=off
  bram_wr_out_sim : Subsystem  mask{we_enable=0, ram_sel=3, add_vec=512, data_in=32}
      mask prompts: we_enable "Write enable"; ram_sel "RAM selector (1 = Re; 2 = Im; 3 = both)"; add_vec "RAM address"; data_in "Data in"
  bram_wr_reg : xps_library/software register  Tag=xps:sw_reg  io_dir=From Processor  arith_type=Unsigned  bitwidth=32  bin_pt=0  sample_period=1  gw_name=seti_ct_xaui_sys_tvg_out_bram_wr_reg_user_data_out
  data_in : xbsIndex_r3/Slice  mode=Lower Bit Location + Width  nbits=18  bit1=0  base1=MSB of Input  bit0=0  base0=LSB of Input  boolean_output=off  explicit_period=on  period=1  dbl_ovrd=off
  ram_im : xps_library/Shared BRAM  Tag=xps:bram  arith_type="Signed  (2's comp)"  addr_width=11  data_width=32  data_bin_pt=0  init_vals=[1:2^11]  sample_rate=1
  ram_re : xps_library/Shared BRAM  Tag=xps:bram  arith_type="Signed  (2's comp)"  addr_width=11  data_width=32  data_bin_pt=0  init_vals=[1:2^11]  sample_rate=1
  thr_cpu_ctrl_sim : Subsystem  mask{tvg_skip=1, tvg_stall=2, tvg_length=5}
      mask prompts: tvg_skip "Skip"; tvg_stall "Stall"; tvg_length "Length"
      mask help:
      | Mux Data for CT and FFT Syncs:
      |
      | 0 -> Interchip Connection
      | 1 -> User Generated External Sync
      | 2 -> Periodic Sync Generator
      | 3 -> Periodic Sync Generator (Same as 2)
      |
      | Mux Data for CT and FFT Inputs:
      |
      | 0 -> Interchip Connection
      | 1 -> Test Vector Generator (TVG)
      | 2 -> All Zeroes (0's)
      | 3 -> All Ones (1's)
  tvg : Subsystem  mask(Test Vector Generator(TVG)){tvg_skip=1, tvg_stall=1, tvg_length=512}
      mask prompts: tvg_skip "Skip"; tvg_stall "Stall"; tvg_length "Length"
  tvg_ctrl : xps_library/software register  Tag=xps:sw_reg  io_dir=From Processor  arith_type=Unsigned  bitwidth=32  bin_pt=0  sample_period=1  gw_name=seti_ct_xaui_sys_tvg_out_tvg_ctrl_user_data_out
  re_out : Outport
  im_out : Outport  Port=2
  wires:
  tvg_ctrl/1 -> tvg/1(In1)
  tvg/1(Out1) -> add mux/2, Gateway Out7/1
  Constant3/1 -> RAM select mux/2
  RAM select mux/1 -> RAM sel  Re (0)/1, RAM sel Im (1)/1
  RAM sel  Re (0)/1 -> ram_re/3
  WE/1 -> Delay/1
  Gateway Out1/1 -> Scope1/1
  Gateway Out2/1 -> Scope1/2
  thr_cpu_ctrl_sim/1(out) -> tvg_ctrl/1
  bram_wr_reg/1 -> data_in/1, add_vec/1, RAM_sel/1, WE/1
  add_vec/1 -> Delay2/1
  RAM_sel/1 -> Delay1/1
  add mux/1 -> ram_im/1, ram_re/1, Gateway Out8/1
  data_in/1 -> Delay3/1
  RAM sel Im (1)/1 -> ram_im/3
  ram_re/1 -> Gateway Out1/1, re_out/1
  ram_im/1 -> Gateway Out2/1, im_out/1
  bram_wr_out_sim/1(Out1) -> bram_wr_reg/1
  Gateway Out3/1 -> Scope2/1
  Gateway Out4/1 -> Scope2/2
  Gateway Out5/1 -> Scope2/3
  Gateway Out6/1 -> Scope2/4
  Delay/1 -> Gateway Out3/1, add mux/1, RAM select mux/1
  Delay1/1 -> Gateway Out4/1, RAM select mux/3
  Delay2/1 -> Gateway Out5/1, add mux/3
  Delay3/1 -> Gateway Out6/1, Delay4/1
  Gateway Out7/1 -> Scope3/1
  Gateway Out8/1 -> Scope3/2
  Delay4/1 -> ram_re/2, ram_im/2

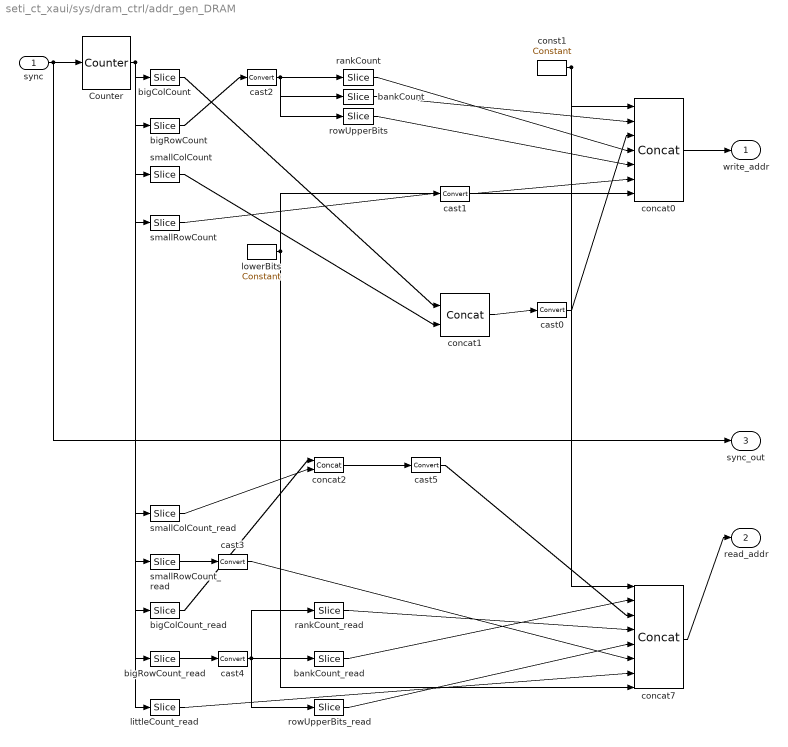
== system seti_ct_xaui/sys/dram_ctrl/addr_gen_DRAM ==
  sync : Inport  Port=1  LatchInput=off
  Counter : xbsIndex_r3/Counter  cnt_type=Free Running  n_bits=counterBitwidth  bin_pt=0  arith_type=Unsigned  start_count=0  cnt_to=Inf  cnt_by_val=1  operation=Up  explicit_period=off  period=1  load_pin=off  rst=on  en=off  dbl_ovrd=off  show_param=off  use_rpm=on  gen_core=off
      settings: xl_area=[0, 0, 0, 0, 0, 0, 0]
  bankCount : xbsIndex_r3/Slice  mode=Upper Bit Location + Width  nbits=2  bit1=-1  base1=MSB of Input  bit0=0  base0=LSB of Input  boolean_output=off  explicit_period=off  period=1  dbl_ovrd=off
  bankCount_read : xbsIndex_r3/Slice  mode=Upper Bit Location + Width  nbits=2  bit1=-1  base1=MSB of Input  bit0=0  base0=LSB of Input  boolean_output=off  explicit_period=off  period=1  dbl_ovrd=off
  bigColCount : xbsIndex_r3/Slice  mode=Lower Bit Location + Width  nbits=bigColBits  bit1=0  base1=MSB of Input  bit0=smallRowBits+smallColBits+bigRowBits  base0=LSB of Input  boolean_output=off  explicit_period=off  period=1  dbl_ovrd=off
  bigColCount_read : xbsIndex_r3/Slice  mode=Lower Bit Location + Width  nbits=bigColBits  bit1=0  base1=MSB of Input  bit0=bigRowBits+2  base0=LSB of Input  boolean_output=off  explicit_period=off  period=1  dbl_ovrd=off
  bigRowCount : xbsIndex_r3/Slice  mode=Lower Bit Location + Width  nbits=bigRowBits  bit1=0  base1=MSB of Input  bit0=smallRowBits+smallColBits  base0=LSB of Input  boolean_output=off  explicit_period=off  period=1  dbl_ovrd=off
  bigRowCount_read : xbsIndex_r3/Slice  mode=Lower Bit Location + Width  nbits=bigRowBits  bit1=0  base1=MSB of Input  bit0=2  base0=LSB of Input  boolean_output=off  explicit_period=off  period=1  dbl_ovrd=off
  cast0 : xbsIndex_r3/Convert  arith_type=Unsigned  n_bits=14  bin_pt=0  quantization=Truncate  overflow=Wrap  latency=0  explicit_period=off  period=1  dbl_ovrd=off  show_param=off  inserted_by_tool=off  pipeline=off
      settings: xl_area=[0, 0, 0, 0, 0, 0, 0]
  cast1 : xbsIndex_r3/Convert  arith_type=Unsigned  n_bits=6  bin_pt=0  quantization=Truncate  overflow=Wrap  latency=0  explicit_period=off  period=1  dbl_ovrd=off  show_param=off  inserted_by_tool=off  pipeline=off
      settings: xl_area=[0, 0, 0, 0, 0, 0, 0]
  cast2 : xbsIndex_r3/Convert  arith_type=Unsigned  n_bits=7  bin_pt=0  quantization=Truncate  overflow=Wrap  latency=0  explicit_period=off  period=1  dbl_ovrd=off  show_param=off  inserted_by_tool=off  pipeline=off
      settings: xl_area=[0, 0, 0, 0, 0, 0, 0]
  cast3 : xbsIndex_r3/Convert  arith_type=Unsigned  n_bits=4  bin_pt=0  quantization=Truncate  overflow=Wrap  latency=0  explicit_period=off  period=1  dbl_ovrd=off  show_param=off  inserted_by_tool=off  pipeline=off
      settings: xl_area=[0, 0, 0, 0, 0, 0, 0]
  cast4 : xbsIndex_r3/Convert  arith_type=Unsigned  n_bits=7  bin_pt=0  quantization=Truncate  overflow=Wrap  latency=0  explicit_period=off  period=1  dbl_ovrd=off  show_param=off  inserted_by_tool=off  pipeline=off
      settings: xl_area=[0, 0, 0, 0, 0, 0, 0]
  cast5 : xbsIndex_r3/Convert  arith_type=Unsigned  n_bits=14  bin_pt=0  quantization=Truncate  overflow=Wrap  latency=0  explicit_period=off  period=1  dbl_ovrd=off  show_param=off  inserted_by_tool=off  pipeline=off
      settings: xl_area=[0, 0, 0, 0, 0, 0, 0]
  concat0 : xbsIndex_r3/Concat  num_inputs=7  explicit_period=off  period=1  dbl_ovrd=off
  concat1 : xbsIndex_r3/Concat  num_inputs=2  explicit_period=off  period=1  dbl_ovrd=off
  concat2 : xbsIndex_r3/Concat  num_inputs=2  explicit_period=off  period=1  dbl_ovrd=off
  concat7 : xbsIndex_r3/Concat  num_inputs=8  explicit_period=off  period=1  dbl_ovrd=off
  const1 : xbsIndex_r3/Constant  const=0  equ=P=C  arith_type=Unsigned  n_bits=2  bin_pt=0  opselect=C  inp2=PCIN>>17  opr=+  inp1=P  carry=CIN  iostate=0  explicit_period=on  period=1  dbl_ovrd=off
  littleCount_read : xbsIndex_r3/Slice  mode=Lower Bit Location + Width  nbits=2  bit1=0  base1=MSB of Input  bit0=0  base0=LSB of Input  boolean_output=off  explicit_period=off  period=1  dbl_ovrd=off
  lowerBits : xbsIndex_r3/Constant  const=0  equ=P=C  arith_type=Unsigned  n_bits=3  bin_pt=0  opselect=C  inp2=PCIN>>17  opr=+  inp1=P  carry=CIN  iostate=0  explicit_period=on  period=1  dbl_ovrd=off
  rankCount : xbsIndex_r3/Slice  mode=Upper Bit Location + Width  nbits=1  bit1=0  base1=MSB of Input  bit0=0  base0=LSB of Input  boolean_output=off  explicit_period=off  period=1  dbl_ovrd=off
  rankCount_read : xbsIndex_r3/Slice  mode=Upper Bit Location + Width  nbits=1  bit1=0  base1=MSB of Input  bit0=0  base0=LSB of Input  boolean_output=off  explicit_period=off  period=1  dbl_ovrd=off
  rowUpperBits : xbsIndex_r3/Slice  mode=Lower Bit Location + Width  nbits=4  bit1=0  base1=MSB of Input  bit0=0  base0=LSB of Input  boolean_output=off  explicit_period=off  period=1  dbl_ovrd=off
  rowUpperBits_read : xbsIndex_r3/Slice  mode=Lower Bit Location + Width  nbits=4  bit1=0  base1=MSB of Input  bit0=0  base0=LSB of Input  boolean_output=off  explicit_period=off  period=1  dbl_ovrd=off
  smallColCount : xbsIndex_r3/Slice  mode=Lower Bit Location + Width  nbits=smallColBits  bit1=0  base1=MSB of Input  bit0=smallRowBits  base0=LSB of Input  boolean_output=off  explicit_period=off  period=1  dbl_ovrd=off
  smallColCount_read : xbsIndex_r3/Slice  mode=Lower Bit Location + Width  nbits=smallColBits  bit1=0  base1=MSB of Input  bit0=bigRowBits+bigColBits+smallRowBits  base0=LSB of Input  boolean_output=off  explicit_period=off  period=1  dbl_ovrd=off
  smallRowCount : xbsIndex_r3/Slice  mode=Lower Bit Location + Width  nbits=smallRowBits  bit1=0  base1=MSB of Input  bit0=0  base0=LSB of Input  boolean_output=off  explicit_period=off  period=1  dbl_ovrd=off
  smallRowCount_read : xbsIndex_r3/Slice  mode=Lower Bit Location + Width  nbits=smallRowBits-2  bit1=0  base1=MSB of Input  bit0=bigRowBits+bigColBits+2  base0=LSB of Input  boolean_output=off  explicit_period=off  period=1  dbl_ovrd=off
  write_addr : Outport
  read_addr : Outport  Port=2
  sync_out : Outport  Port=3
  wires:
  Counter/1 -> bigColCount/1, smallColCount/1, bigColCount_read/1, smallColCount_read/1, smallRowCount/1, bigRowCount/1, smallRowCount_read/1, bigRowCount_read/1, littleCount_read/1
  bigColCount/1 -> concat1/1
  smallColCount/1 -> concat1/2
  concat1/1 -> cast0/1
  smallColCount_read/1 -> concat2/2
  bigColCount_read/1 -> concat2/1
  concat2/1 -> cast5/1
  sync/1 -> Counter/1, sync_out/1
  lowerBits/1 -> concat0/7, concat7/8
  cast0/1 -> concat0/3
  cast1/1 -> concat0/6
  rankCount/1 -> concat0/4
  smallRowCount/1 -> cast1/1
  rowUpperBits/1 -> concat0/5
  bankCount/1 -> concat0/2
  const1/1 -> concat0/1, concat7/1
  bigRowCount/1 -> cast2/1
  cast2/1 -> bankCount/1, rankCount/1, rowUpperBits/1
  concat0/1 -> write_addr/1
  smallRowCount_read/1 -> cast3/1
  bigRowCount_read/1 -> cast4/1
  cast4/1 -> rankCount_read/1, bankCount_read/1, rowUpperBits_read/1
  concat7/1 -> read_addr/1
  bankCount_read/1 -> concat7/2
  cast5/1 -> concat7/3
  rankCount_read/1 -> concat7/4
  rowUpperBits_read/1 -> concat7/5
  cast3/1 -> concat7/6
  littleCount_read/1 -> concat7/7

== system seti_ct_xaui/sys/dram_ctrl/cmdAck1 ==
  in : Inport  Port=1  LatchInput=off
  Scope : Scope
  big_negedge : Subsystem
  gpio : xps_library/gpio  Tag=xps:gpio  io_group=BEE2_usr:led  io_dir=out  arith_type=Unsigned  bitwidth=1  bin_pt=0  bit_index=1  sample_period=1  use_single_ended=off  use_ddr=off  reg_iob=on  reg_clk_phase=0  termination=None
  wires:
  gpio/1 -> Scope/1
  in/1 -> big_negedge/1(in)
  big_negedge/1(pulse) -> gpio/1

== system seti_ct_xaui/sys/dram_ctrl/cmdAck2 ==
  in : Inport  Port=1  LatchInput=off
  Scope : Scope
  big_negedge : Subsystem
  gpio : xps_library/gpio  Tag=xps:gpio  io_group=BEE2_usr:led  io_dir=out  arith_type=Unsigned  bitwidth=1  bin_pt=0  bit_index=2  sample_period=1  use_single_ended=off  use_ddr=off  reg_iob=off  reg_clk_phase=0  termination=None
  wires:
  in/1 -> big_negedge/1(in)
  big_negedge/1(pulse) -> gpio/1
  gpio/1 -> Scope/1
